simulink model "c28035blink_cla"  (R2021b)
settings: Solver=FixedStepDiscrete  StartTime=0.0  StopTime=10.0  FixedStep=.5  RelTol=1e-3  EnableMultiTasking=on
libraries: c2806xlib x2, c2000lib x1, demo_controls x1
settings Model: Creator=The MathWorks, Inc.  LastModifiedBy=The MathWorks, Inc.
settings SolverCC: AlgebraicLoopSolver=TrustRegion
settings DataIOCC: LimitDataPoints=on  SaveFormat=Array  SaveOutput=off  SaveTime=off  ReturnWorkspaceOutputs=off
settings OptimizationCC: DefaultParameterBehavior=Inlined  DefaultUnderspecifiedDataType=single  InlineInvariantSignals=on  BufferReuse=off  ExpressionDepthLimit=2147483647  InitFltsAndDblsToZero=on  NoFixptDivByZeroProtection=on  EfficientFloat2IntCast=on  EfficientMapNaN2IntZero=off  LifeSpan=1  MaxStackSize=512  EfficientTunableParamExpr=on
settings DebuggingCC: UnderspecifiedInitializationDetection=Classic  MergeDetectMultiDrivingBlocksExec=none  SolverPrmCheckMsg=warning  MultiTaskDSMMsg=none  MultiTaskCondExecSysMsg=none  FcnCallInpInsideContextMsg=warning  AllowSymbolicDim=off  StateNameClashWarn=warning  SFUnexpectedBacktrackingDiag=warning  SFNoUnconditionalDefaultTransitionDiag=warning  SFExecutionAtInitializationDiag=none  SFMachineParentedDataDiag=warning  ArithmeticOperatorsInVariantConditions=warning
settings HardwareCC: ProdBitPerChar=16  ProdBitPerInt=16  ProdBitPerPointer=32  ProdBitPerSizeT=32  ProdBitPerPtrDiffT=32  ProdLargestAtomicInteger=Integer  ProdLargestAtomicFloat=None  ProdWordSize=16  ProdHWDeviceType=Texas Instruments->C2000
settings ModelReferenceCC: PropagateSignalLabelsOutOfModel=off
settings SFSimCC: SimUseLocalCustomCode=off  MATLABDynamicMemAlloc=off  CustomCodeUndefinedFunction=UseInterfaceOnly
settings RTWCC: Description=Embedded Coder  SystemTargetFile=ert.tlc  HardwareBoard=TI Piccolo F2803x  TemplateMakefile=ert_default_tmf  GenerateReport=on  RTWUseLocalCustomCode=off  Toolchain=Texas Instruments Code Composer Studio (C2000)  BuildConfiguration=Debug  IncludeHyperlinkInReport=on  LaunchReport=on  GenerateTraceInfo=on  GenerateTraceReport=on  GenerateTraceReportSl=on  GenerateTraceReportSf=on  GenerateTraceReportEml=on
settings CodeAppCC: IgnoreCustomStorageClasses=off  CustomSymbolStrType=$N$R$M  StateflowObjectComments=on  InternalIdentifier=Classic
settings ERTTargetCC: MultiwordLength=2048  ExtModeStaticAllocSize=2048  InlinedParameterPlacement=NonHierarchical  ConvertIfToSwitch=off  SuppressUnreachableDefaultCases=off
settings ConfigComp: CovMetricSettings=dw  CovSaveCumulativeToWorkspaceVar=on  CovSaveSingleToWorkspaceVar=on  CovExternalEMLEnable=off  CovSFcnEnable=off

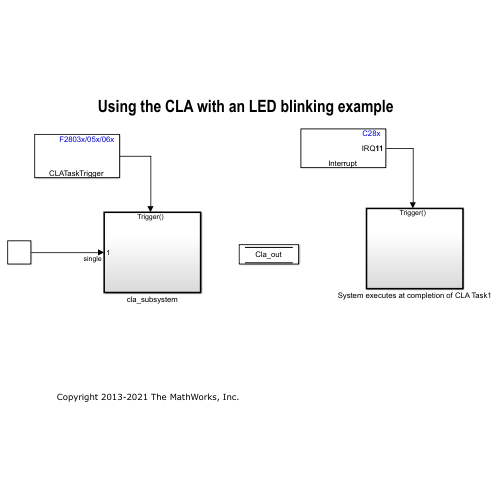
[thumbnail: Simulink's stored preview of the top-level diagram]
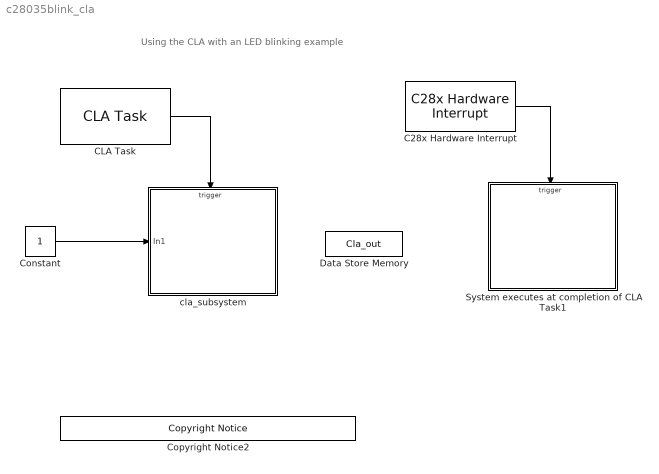
== system c28035blink_cla ==
  note: Using the CLA with an LED blinking example
  C28x Hardware Interrupt : c2000lib/Scheduling/C28x Hardware Interrupt  irqnumbers=[11]  pienumbers=[1]  irqpriorities=[30]  irqpreempts=[0]  showinput=off  dspchiptype=C280X
      settings: SourceProductBaseCode=TIC2000
  CLA Task : c2806xlib/CLA Task  taskNumber=1  intSource=Software  sampleTime=0.5  claType=0  softTrigSelected=1  enableInterrupt=on
      settings: SourceProductBaseCode=TIC2000
  Constant : Constant  OutDataTypeStr=single  SampleTime=0.5
  Copyright Notice2 : demo_controls/Copyright Notice  year=2013  prod=tic2000
      settings: SourceProductBaseCode=ME
  Data Store Memory : DataStoreMemory  DataStoreName=Cla_out  EmbeddedSignalClassName=tic2000demospkg.Signal  ShowAdditionalParam=off  OutDataTypeStr=boolean
  System executes at completion of CLA Task1 : Subsystem  TreatAsAtomicUnit=on  RTWFcnName=Cla1Task1  RTWFileName=sample_cla
      settings: RTWFileNameOpts=User specified  RTWMemSecFuncInitTerm=Default  RTWMemSecFuncExecute=Default  RTWMemSecDataInternal=Default
  cla_subsystem : Subsystem  TreatAsAtomicUnit=on  RTWFcnName=Cla1Task1  RTWFileName=sample_cla
      settings: RTWSystemCode=Inline  RTWFileNameOpts=User specified  RTWMemSecFuncInitTerm=Default  RTWMemSecFuncExecute=Default  RTWMemSecDataInternal=Default
  wires:
  Constant/1 -> cla_subsystem/1(In1)
  CLA Task/1 -> cla_subsystem/Trigger
  C28x Hardware Interrupt/1 -> System executes at completion of CLA Task1/Trigger

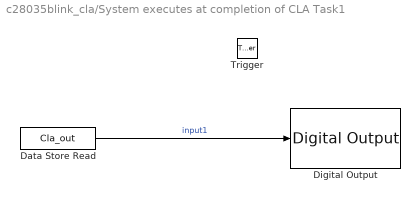
== system c28035blink_cla/System executes at completion of CLA Task1 ==
  Trigger : TriggerPort  TriggerType=function-call  VariantControl=Variant  PortDimensions=1
  Data Store Read : DataStoreRead  DataStoreName=Cla_out  IndexOptions=Index vector (dialog)  Indices=1  OutputSizes=1
  Digital Output : c2806xlib/Digital Output  GPIO_Number=GPIO32~GPIO39  GPIO_Bit0=off  GPIO_BIT0_Toggle=off  GPIO_Bit1=off  GPIO_BIT1_Toggle=off  GPIO_Bit2=on  GPIO_BIT2_Toggle=off  GPIO_Bit3=off  GPIO_BIT3_Toggle=off  GPIO_Bit4=off  GPIO_BIT4_Toggle=off  GPIO_Bit5=off  GPIO_BIT5_Toggle=off  GPIO_Bit6=off  GPIO_BIT6_Toggle=off  GPIO_Bit7=off  GPIO_BIT7_Toggle=off
      settings: SourceProductBaseCode=TIC2000
  wires:
  Data Store Read/1 -> Digital Output/1  "input1"

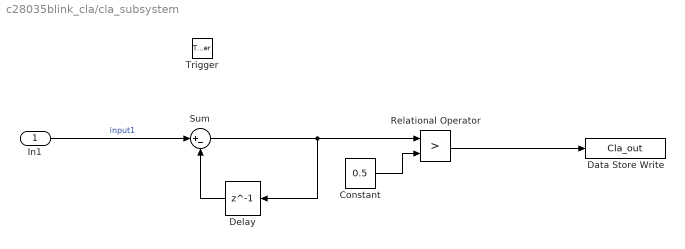
== system c28035blink_cla/cla_subsystem ==
  In1 : Inport  OutDataTypeStr=single
  Trigger : TriggerPort  TriggerType=function-call  VariantControl=Variant  PortDimensions=1
  Constant : Constant  Value=0.5  OutDataTypeStr=single
  Data Store Write : DataStoreWrite  DataStoreName=Cla_out  IndexOptions=Index vector (dialog)  Indices=1  OutputSizes=1
  Delay : Delay  DelayLength=1  InitialCondition=0  StateName=fb_delay  EmbeddedSignalClassName=tic2000demospkg.Signal
  Relational Operator : RelationalOperator  Operator=>  OutDataTypeStr=boolean  RndMeth=Nearest
  Sum : Sum  Inputs=|+-  AccumDataTypeStr=single  RndMeth=Round
  wires:
  In1/1 -> Sum/1  "input1"
  Delay/1 -> Sum/2
  Sum/1 -> Delay/1, Relational Operator/1
  Constant/1 -> Relational Operator/2
  Relational Operator/1 -> Data Store Write/1
